simulink model "OMSv1_2x"  (Simulink 6.5)
settings: Solver=ode4  SolverMode=SingleTasking  StartTime=0.0  StopTime=5  FixedStep=0.001  MaxStep=0.001  RelTol=1e-3  AbsTol=1e-3
undefined symbols (not defined in the file): alexlaw, bs_onoff, bs_scale, bsfsacrit, bsfsvcrit, cnsgain, fs_onoff, fs_scale, fsdelaycalc, ltdrk, phasicgain, pmcgain, pmctau2, pmctau3, saccsw, spgain, tonicgain, tvrD, tvrN
libraries: simulink_extras x37
(part 3 of 5)

== system OMSv1_2x/OMS v1.2  07/21/05/IM CN-LMLN/Saccade Enable/prolong ==
  note: init Q = 0
  note: Stretch the duration of an input pulse, latching it at its value at pulse onset.
  note: The one integration step delay before the S&H block's S/H (bottom) input insures
      | that the input value to be latched is available to theS&H block's top input
      | before the S&H block tries to 'hold'.
  note: The start of the input pulse causes the value on input 1 to be held starting when the leading
      | edge occurs, and this value remains latched until 'delay' seconds after the pulse ends (trailing edge).
  note: 11/22/99
  note: init = 0
  note: init = 0
  value(in) : Inport
  " x/1000" : Constant  Orientation=up  Value=0.001
  Latch1 : simulink_extras/Flip Flops/S-R Flip-Flop  SystemSampleTime=-1  initial_condition=0
  Product : Product  SaturateOnIntegerOverflow=on  RndMeth=Zero  InputSameDT=on
  SampHold?2 : Subsystem
      mask Display: disp('S=L\nH=H')
  Terminator : Terminator
  Variable Transport Delay : VariableTransportDelay  MaximumDelay=10  MaximumPoints=prolong_buffersize
  leading edge detect : Subsystem
      mask Display: disp('Leading\nEdge Det')
  loop breaker2 : Memory
  stretch : Constant  Value=prolong
  trailing edge detect : Subsystem
      mask Display: disp('Trailing\nEdge Det')
  value(out) : Outport  InitialOutput=0
  wires:
  value(in)/1 -> leading edge detect/1(in_1), trailing edge detect/1(in_1), SampHold?2/1(Input)
  Variable Transport Delay/1 -> Latch1/2
  trailing edge detect/1(out_1) -> Variable Transport Delay/1
  leading edge detect/1(out_1) -> Latch1/1
  Latch1/1 -> loop breaker2/1
  SampHold?2/1(output) -> value(out)/1
  loop breaker2/1 -> SampHold?2/2(S/H?)
  stretch/1 -> Product/1
  Product/1 -> Variable Transport Delay/2
  " x/1000"/1 -> Product/2
  Latch1/2 -> Terminator/1

== system OMSv1_2x/OMS v1.2  07/21/05/IM CN-LMLN/Saccade Enable/trailing edge detect ==
  note: trailing edge detection
  note: It is also possible to remove the SIGNUM function
      | and the '==', and replace them with a simple
      | switch with a threshold of (say) 150 or so.
  PG : Inport
  Abs : Abs  SaturateOnIntegerOverflow=on
  Derivative : Derivative
  Relational Operator : RelationalOperator  Operator===  InputSameDT=on
  Sign : Signum
  Threshold 1 : Constant  Value=-1
  Latch R : Outport  InitialOutput=0
  wires:
  PG/1 -> Abs/1
  Relational Operator/1 -> Latch R/1
  Threshold 1/1 -> Relational Operator/2
  Sign/1 -> Relational Operator/1
  Derivative/1 -> Sign/1
  Abs/1 -> Derivative/1

== system OMSv1_2x/OMS v1.2  07/21/05/IM CN-LMLN/Saccade Motor Commmand/TCHNG Override ==
  note: (FF init state: Q=1)
  note: * Leading Edge of input ENABLEs output
  note: Operation:
  note: *FS Enabling is initially DISABLED
  note: * Output of TIMER circuit DISABLES output
  note: TCHNG Override
  "[tchng]" : Inport
  timer dur : Inport  Orientation=up  Port=2
  Latch1 : simulink_extras/Flip Flops/S-R Flip-Flop  SystemSampleTime=-1  initial_condition=1
  Terminator : Terminator
  event timer2 : Subsystem
      mask Display: disp('Event\nTimer2')
  leading edge detect : Subsystem
      mask Display: disp('Leading\nEdge Det')
  tchng sw : Outport  InitialOutput=0
  wires:
  "[tchng]"/1 -> leading edge detect/1(in_1), event timer2/1(_PG)
  timer dur/1 -> event timer2/2(_timer value (port))
  event timer2/1(out_1) -> Latch1/1
  leading edge detect/1(out_1) -> Latch1/2
  Latch1/1 -> tchng sw/1
  Latch1/2 -> Terminator/1

== system OMSv1_2x/OMS v1.2  07/21/05/IM CN-LMLN/Saccade Motor Commmand/Voluntary Saccade Switch ==
  note: Voluntary Saccade Switch
  note: move this outpt
      | to top switch
  note: last mod:
      | 02/26/01
  "[fphmag]" : Inport
  "[sacenab]" : Inport  Port=2
  "[fsorbs30]" : Inport  Port=3
  (0.5)1 : Switch  Threshold=.5  SaturateOnIntegerOverflow=on  InputSameDT=on
  (0.5)2 : Switch  Threshold=.5  SaturateOnIntegerOverflow=on  InputSameDT=on
  (0.5)3 : Switch  Threshold=.5  SaturateOnIntegerOverflow=on  InputSameDT=on
  Logical Operator4 : Logic  Operator=NOT  Inputs=1
  Logical Operator6 : Logic  Operator=OR
  oppose3 : Constant  Orientation=left  Value=0
  saccsw : Constant  Orientation=left  Value=saccsw
  "[vsmc]" : Outport  InitialOutput=0
  sacenab/0 : Outport  Port=2  InitialOutput=0
  wires:
  "[fphmag]"/1 -> (0.5)2/1
  "[fsorbs30]"/1 -> Logical Operator4/1
  Logical Operator4/1 -> Logical Operator6/2
  (0.5)2/1 -> (0.5)3/1
  Logical Operator6/1 -> sacenab/0/1
  saccsw/1 -> (0.5)2/3, (0.5)2/2, (0.5)1/2, (0.5)1/3
  "[sacenab]"/1 -> (0.5)1/1, (0.5)3/2
  (0.5)1/1 -> Logical Operator6/1
  oppose3/1 -> (0.5)3/3
  (0.5)3/1 -> "[vsmc]"/1

== system OMSv1_2x/OMS v1.2  07/21/05/IM CN-LMLN/Sampled Target Reconstruction/Boolify ==
  In1 : Inport
  Abs2 : Abs  SaturateOnIntegerOverflow=on
  direction1 : Signum
  Out1 : Outport  InitialOutput=0
  wires:
  direction1/1 -> Out1/1
  In1/1 -> Abs2/1
  Abs2/1 -> direction1/1

== system OMSv1_2x/OMS v1.2  07/21/05/IM CN-LMLN/Sampled Target Reconstruction/Boolify1 ==
  In1 : Inport
  Abs2 : Abs  SaturateOnIntegerOverflow=on
  direction1 : Signum
  Out1 : Outport  InitialOutput=0
  wires:
  Abs2/1 -> direction1/1
  In1/1 -> Abs2/1
  direction1/1 -> Out1/1

== system OMSv1_2x/OMS v1.2  07/21/05/IM CN-LMLN/Sampled Target Reconstruction/DZ 0.3 ==
  note: We just output zero when the dead zone is in effect, and leave the
      |  output alone the rest of the time.
  note: This block is a better implementation of a dead zone than  the
      | block supplied by SIMULINK, because here we don't _subtract_
      | the dead zone from the rest of output.
  in_1 : Inport
  Abs : Abs  Orientation=down  SaturateOnIntegerOverflow=on
  Relational Operator : RelationalOperator  InputSameDT=on
  Switch6 : Switch  Threshold=.5  SaturateOnIntegerOverflow=on  InputSameDT=on
  dead zone : Constant  Orientation=up  Value=.3
  pos (deg) criterion1 : Constant  Orientation=left  Value=0
  out_1 : Outport  InitialOutput=0
  wires:
  Relational Operator/1 -> Switch6/2
  dead zone/1 -> Relational Operator/2
  pos (deg) criterion1/1 -> Switch6/3
  Abs/1 -> Relational Operator/1
  in_1/1 -> Abs/1, Switch6/1
  Switch6/1 -> out_1/1

== system OMSv1_2x/OMS v1.2  07/21/05/IM CN-LMLN/Sampled Target Reconstruction/SampHold? ==
  note: When "S/H?" is HIGH, then "Input" is switched directly to the
      | output ("sample").  When "S/H?" is LOW, the current output is
      | maintained ("hold").
  Input : Inport
  S/H? : Inport  Port=2
  Memory : Memory  Orientation=left
  Sign : Signum
  Switch2 : Switch  Threshold=0.5  SaturateOnIntegerOverflow=on  InputSameDT=on
  output : Outport  InitialOutput=0
  wires:
  S/H?/1 -> Sign/1
  Sign/1 -> Switch2/2
  Input/1 -> Switch2/1
  Switch2/1 -> output/1, Memory/1
  Memory/1 -> Switch2/3

== system OMSv1_2x/OMS v1.2  07/21/05/IM CN-LMLN/Sampled Target Reconstruction/leading edge detect1 ==
  note: leading edge detection
  in_1 : Inport
  Abs : Abs  SaturateOnIntegerOverflow=on
  Derivative : Derivative
  Relational Operator : RelationalOperator  Operator===  InputSameDT=on
  Sign : Signum
  Threshold 1 : Constant
  out_1 : Outport  InitialOutput=0
  wires:
  Abs/1 -> Derivative/1
  Derivative/1 -> Sign/1
  Sign/1 -> Relational Operator/1
  Threshold 1/1 -> Relational Operator/2
  Relational Operator/1 -> out_1/1
  in_1/1 -> Abs/1

== system OMSv1_2x/OMS v1.2  07/21/05/IM CN-LMLN/Sampled Target Reconstruction/leading edge detect2 ==
  note: leading edge detection
  in_1 : Inport
  Abs : Abs  SaturateOnIntegerOverflow=on
  Derivative : Derivative
  Relational Operator : RelationalOperator  Operator===  InputSameDT=on
  Sign : Signum
  Threshold 1 : Constant
  out_1 : Outport  InitialOutput=0
  wires:
  in_1/1 -> Abs/1
  Relational Operator/1 -> out_1/1
  Threshold 1/1 -> Relational Operator/2
  Sign/1 -> Relational Operator/1
  Derivative/1 -> Sign/1
  Abs/1 -> Derivative/1

== system OMSv1_2x/OMS v1.2  07/21/05/IM CN-LMLN/Sampled Target Reconstruction/prolong ==
  note: init = 0
  note: init = 0
  note: 11/22/99
  note: The start of the input pulse causes the value on input 1 to be held starting when the leading
      | edge occurs, and this value remains latched until 'delay' seconds after the pulse ends (trailing edge).
  note: The one integration step delay before the S&H block's S/H (bottom) input insures
      | that the input value to be latched is available to theS&H block's top input
      | before the S&H block tries to 'hold'.
  note: Stretch the duration of an input pulse, latching it at its value at pulse onset.
  note: init Q = 0
  value(in) : Inport
  " x/1000" : Constant  Orientation=up  Value=0.001
  Latch1 : simulink_extras/Flip Flops/S-R Flip-Flop  SystemSampleTime=-1  initial_condition=0
  Product : Product  SaturateOnIntegerOverflow=on  RndMeth=Zero  InputSameDT=on
  SampHold?2 : Subsystem
      mask Display: disp('S=L\nH=H')
  Terminator : Terminator
  Variable Transport Delay : VariableTransportDelay  MaximumDelay=10  MaximumPoints=prolong_buffersize
  leading edge detect : Subsystem
      mask Display: disp('Leading\nEdge Det')
  loop breaker2 : Memory
  stretch : Constant  Value=prolong
  trailing edge detect : Subsystem
      mask Display: disp('Trailing\nEdge Det')
  value(out) : Outport  InitialOutput=0
  wires:
  " x/1000"/1 -> Product/2
  Product/1 -> Variable Transport Delay/2
  stretch/1 -> Product/1
  loop breaker2/1 -> SampHold?2/2(S/H?)
  SampHold?2/1(output) -> value(out)/1
  Latch1/1 -> loop breaker2/1
  leading edge detect/1(out_1) -> Latch1/1
  trailing edge detect/1(out_1) -> Variable Transport Delay/1
  Variable Transport Delay/1 -> Latch1/2
  value(in)/1 -> SampHold?2/1(Input), trailing edge detect/1(in_1), leading edge detect/1(in_1)
  Latch1/2 -> Terminator/1

== system OMSv1_2x/OMS v1.2  07/21/05/IM CN-LMLN/Sampled Target Reconstruction/prolong1 ==
  note: init Q = 0
  note: Stretch the duration of an input pulse, latching it at its value at pulse onset.
  note: The one integration step delay before the S&H block's S/H (bottom) input insures
      | that the input value to be latched is available to theS&H block's top input
      | before the S&H block tries to 'hold'.
  note: The start of the input pulse causes the value on input 1 to be held starting when the leading
      | edge occurs, and this value remains latched until 'delay' seconds after the pulse ends (trailing edge).
  note: 11/22/99
  note: init = 0
  note: init = 0
  value(in) : Inport
  " x/1000" : Constant  Orientation=up  Value=0.001
  Latch1 : simulink_extras/Flip Flops/S-R Flip-Flop  SystemSampleTime=-1  initial_condition=0
  Product : Product  SaturateOnIntegerOverflow=on  RndMeth=Zero  InputSameDT=on
  SampHold?2 : Subsystem
      mask Display: disp('S=L\nH=H')
  Terminator : Terminator
  Variable Transport Delay : VariableTransportDelay  MaximumDelay=10  MaximumPoints=prolong_buffersize
  leading edge detect : Subsystem
      mask Display: disp('Leading\nEdge Det')
  loop breaker2 : Memory
  stretch : Constant  Value=prolong
  trailing edge detect : Subsystem
      mask Display: disp('Trailing\nEdge Det')
  value(out) : Outport  InitialOutput=0
  wires:
  value(in)/1 -> leading edge detect/1(in_1), trailing edge detect/1(in_1), SampHold?2/1(Input)
  Variable Transport Delay/1 -> Latch1/2
  trailing edge detect/1(out_1) -> Variable Transport Delay/1
  leading edge detect/1(out_1) -> Latch1/1
  Latch1/1 -> loop breaker2/1
  SampHold?2/1(output) -> value(out)/1
  loop breaker2/1 -> SampHold?2/2(S/H?)
  stretch/1 -> Product/1
  Product/1 -> Variable Transport Delay/2
  " x/1000"/1 -> Product/2
  Latch1/2 -> Terminator/1

== system OMSv1_2x/OMS v1.2  07/21/05/IM CN-LMLN/Sampled Target Reconstruction/prolong2 ==
  note: init = 0
  note: init = 0
  note: 11/22/99
  note: The start of the input pulse causes the value on input 1 to be held starting when the leading
      | edge occurs, and this value remains latched until 'delay' seconds after the pulse ends (trailing edge).
  note: The one integration step delay before the S&H block's S/H (bottom) input insures
      | that the input value to be latched is available to theS&H block's top input
      | before the S&H block tries to 'hold'.
  note: Stretch the duration of an input pulse, latching it at its value at pulse onset.
  note: init Q = 0
  value(in) : Inport
  " x/1000" : Constant  Orientation=up  Value=0.001
  Latch1 : simulink_extras/Flip Flops/S-R Flip-Flop  SystemSampleTime=-1  initial_condition=0
  Product : Product  SaturateOnIntegerOverflow=on  RndMeth=Zero  InputSameDT=on
  SampHold?2 : Subsystem
      mask Display: disp('S=L\nH=H')
  Terminator : Terminator
  Variable Transport Delay : VariableTransportDelay  MaximumDelay=10  MaximumPoints=prolong_buffersize
  leading edge detect : Subsystem
      mask Display: disp('Leading\nEdge Det')
  loop breaker2 : Memory
  stretch : Constant  Value=prolong
  trailing edge detect : Subsystem
      mask Display: disp('Trailing\nEdge Det')
  value(out) : Outport  InitialOutput=0
  wires:
  " x/1000"/1 -> Product/2
  Product/1 -> Variable Transport Delay/2
  stretch/1 -> Product/1
  loop breaker2/1 -> SampHold?2/2(S/H?)
  SampHold?2/1(output) -> value(out)/1
  Latch1/1 -> loop breaker2/1
  leading edge detect/1(out_1) -> Latch1/1
  trailing edge detect/1(out_1) -> Variable Transport Delay/1
  Variable Transport Delay/1 -> Latch1/2
  value(in)/1 -> SampHold?2/1(Input), trailing edge detect/1(in_1), leading edge detect/1(in_1)
  Latch1/2 -> Terminator/1

== system OMSv1_2x/OMS v1.2  07/21/05/IM CN-LMLN/Slip Velocity Reconstruction/DZ 0.5 ==
  note: We just output zero when the dead zone is in effect, and leave the
      |  output alone the rest of the time.
  note: This block is a better implementation of a dead zone than  the
      | block supplied by SIMULINK, because here we don't _subtract_
      | the dead zone from the rest of output.
  in_1 : Inport
  in_2 : Inport  Port=2
  Abs : Abs  Orientation=down  SaturateOnIntegerOverflow=on
  Relational Operator : RelationalOperator  InputSameDT=on
  Switch6 : Switch  Threshold=.5  SaturateOnIntegerOverflow=on  InputSameDT=on
  pos (deg) criterion1 : Constant  Orientation=left  Value=0
  out_1 : Outport  InitialOutput=0
  wires:
  Relational Operator/1 -> Switch6/2
  pos (deg) criterion1/1 -> Switch6/3
  Switch6/1 -> out_1/1
  in_2/1 -> Relational Operator/2
  Abs/1 -> Relational Operator/1
  in_1/1 -> Abs/1, Switch6/1

== system OMSv1_2x/OMS v1.2  07/21/05/IM CN-LMLN/Slip Velocity Reconstruction/Lim 100 ==
  note: This block limits outputs to less than or equal to the "Limit" constant.
      | Inputs greater than "Limit" yield a zero output.
  in_1 : Inport
  Abs : Abs  SaturateOnIntegerOverflow=on
  Limit : Constant  Orientation=up  Value=100
  Product : Product  SaturateOnIntegerOverflow=on  RndMeth=Zero  InputSameDT=on
  Relational Operator : RelationalOperator  Operator=<=  InputSameDT=on
  out_1 : Outport  InitialOutput=0
  wires:
  in_1/1 -> Product/1, Abs/1
  Abs/1 -> Relational Operator/1
  Relational Operator/1 -> Product/2
  Limit/1 -> Relational Operator/2
  Product/1 -> out_1/1

== system OMSv1_2x/OMS v1.2  07/21/05/IM CN-LMLN/Slip Velocity Reconstruction/SampHold?4 ==
  note: When "S/H?" is HIGH, then "Input" is switched directly to the
      | output ("sample").  When "S/H?" is LOW, the current output is
      | maintained ("hold").
  Input : Inport
  S/H? : Inport  Port=2
  Memory : Memory  Orientation=left
  Sign : Signum
  Switch2 : Switch  Threshold=0.5  SaturateOnIntegerOverflow=on  InputSameDT=on
  output : Outport  InitialOutput=0
  wires:
  S/H?/1 -> Sign/1
  Sign/1 -> Switch2/2
  Switch2/1 -> output/1, Memory/1
  Input/1 -> Switch2/1
  Memory/1 -> Switch2/3

== system OMSv1_2x/OMS v1.2  07/21/05/PG w rNI1/PW funct/Good Reset Integrator1 ==
  note: This Resettable integrator won't (incorrectly) integrate the input even
      | when the reset signal is held, unlike the SIMULINK RI, which
      | gives a one time-step error.
  note: reset on either rising
      | edge or level signal
  note: changed 7/22
  note: Using 'state' port, rather than 'output'
      | port to avoid algebraic loop*
  note: *see: www.mathworks.com/access/helpdesk/toolbox/simulink/slref/integrator.html
  input : Inport
  reset? : Inport  Port=2
  initial condition : Inport  Port=3
  Integrator : Integrator  ExternalReset=either  InitialConditionSource=external  ShowStatePort=on
  Logical Operator2 : Logic  Orientation=up  Operator=NOT  Inputs=1
  Product : Product  SaturateOnIntegerOverflow=on  RndMeth=Zero  InputSameDT=on
  Terminator : Terminator
  out_1 : Outport  InitialOutput=0
  wires:
  initial condition/1 -> Integrator/3
  Logical Operator2/1 -> Product/2
  input/1 -> Product/1
  Product/1 -> Integrator/1
  reset?/1 -> Integrator/2, Logical Operator2/1
  Integrator/State -> out_1/1
  Integrator/1 -> Terminator/1

== system OMSv1_2x/OMS v1.2  07/21/05/PG w rNI1/PW funct/Input Switch ==
  mcspl : Inport
  pgw : Inport  Port=2
  Switch2 : Switch  Threshold=0.5  SaturateOnIntegerOverflow=on  InputSameDT=on
  lead/trail edge det : Subsystem
      mask Display: disp('Lead/Trail\nEdge Det')
  mcsw : Outport  InitialOutput=0
  wires:
  mcspl/1 -> Switch2/1, lead/trail edge det/1(in_1)
  pgw/1 -> Switch2/2
  lead/trail edge det/1(out_1) -> Switch2/3
  Switch2/1 -> mcsw/1

== system OMSv1_2x/OMS v1.2  07/21/05/PG w rNI1/RefLatch (Default = 50ms)/trailing edge ==
  note: (FF init state: Q=1)
  note: (Init input: 0)
  note: When the latency period is over, the block is again ENABLED.  ONLY once the latency period is
      | over does the block accept any new input.  (i.e. any input that occurs during the disabled
      |  latency period is ignored)
  note: When input occurs, the block then becomes DISABLED, and remains so for the
      | duration of the latency period (set either via the mask, or by setting "delay" from the command line)
  note: Block operation: it is initially ENABLED, allowing input.
  note: latency period starts with the END of the pulse, rather than the beginning.
  note: (Init input: 1)
  note: (Must see a trailing edge from the
      | signal AS WELL)
  note: This upper branch prevents response
      | to transients caused by the switch
      | toggling states
  in_1 : Inport
  Logical Operator : Logic
  S-R Flip-Flop : simulink_extras/Flip Flops/S-R Flip-Flop  SystemSampleTime=-1  initial_condition=1
  Switch1 : Switch  Threshold=.5  SaturateOnIntegerOverflow=on  InputSameDT=on
  Terminator : Terminator
  Threshold 3 : Constant  Orientation=left  Value=0
  loop breaker : Memory  Orientation=left  X0=1
  refractory period : TransportDelay  DelayTime=(delay)/1000
  trailing edge det : Subsystem
      mask Display: disp('Trailing\nEdge Det')
  trailing edge det1 : Subsystem
      mask Display: disp('Trailing\nEdge Det')
  out_1 : Outport  InitialOutput=0
  wires:
  S-R Flip-Flop/1 -> out_1/1, loop breaker/1
  Logical Operator/1 -> S-R Flip-Flop/2, refractory period/1
  trailing edge det/1(out_1) -> Logical Operator/1
  trailing edge det1/1(out_1) -> Logical Operator/2
  in_1/1 -> Switch1/1, trailing edge det/1(in_1)
  refractory period/1 -> S-R Flip-Flop/1
  loop breaker/1 -> Switch1/2
  Threshold 3/1 -> Switch1/3
  Switch1/1 -> trailing edge det1/1(in_1)
  S-R Flip-Flop/2 -> Terminator/1

== system OMSv1_2x/OMS v1.2  07/21/05/IM CN-LMLN/BS/FS Logic/BS Enable1/BS Timing ==
  note: (FF init state: Q=0)
  note: * Leading Edge of input ENABLEs output
  note: Operation:
  note: *BS Enabling is initially DISABLED
  note: * Output of TIMER circuit DISABLES output
  note: BS Timing
  From  <= [cmpr] : Inport
  timer dur : Inport  Orientation=up  Port=2
  Latch1 : simulink_extras/Flip Flops/S-R Flip-Flop  SystemSampleTime=-1  initial_condition=0
  Terminator : Terminator
  event timer2 : Subsystem
      mask Display: disp('Event\nTimer2')
  leading edge detect : Subsystem
      mask Display: disp('Leading\nEdge Det')
  "[bsenab]" : Outport  InitialOutput=0
  wires:
  From  <= [cmpr]/1 -> leading edge detect/1(in_1), event timer2/1(_PG)
  leading edge detect/1(out_1) -> Latch1/1
  event timer2/1(out_1) -> Latch1/2
  Latch1/1 -> "[bsenab]"/1
  timer dur/1 -> event timer2/2(_timer value (port))
  Latch1/2 -> Terminator/1

== system OMSv1_2x/OMS v1.2  07/21/05/IM CN-LMLN/BS/FS Logic/FS Enable/FS Timing ==
  note: FS Timing
  note: * Output of TIMER circuit DISABLES output
  note: *FS Enabling is initially DISABLED
  note: Operation:
  note: * Leading Edge of input ENABLEs output
  note: (FF init state: Q=0)
  From  <= [cmpr] : Inport
  timer dur : Inport  Orientation=up  Port=2
  Latch1 : simulink_extras/Flip Flops/S-R Flip-Flop  SystemSampleTime=-1  initial_condition=0
  Terminator : Terminator
  event timer2 : Subsystem
      mask Display: disp('Event\nTimer2')
  leading edge detect : Subsystem
      mask Display: disp('Leading\nEdge Det')
  "[fsenab]" : Outport  InitialOutput=0
  wires:
  timer dur/1 -> event timer2/2(_timer value (port))
  Latch1/1 -> "[fsenab]"/1
  event timer2/1(out_1) -> Latch1/2
  leading edge detect/1(out_1) -> Latch1/1
  From  <= [cmpr]/1 -> event timer2/1(_PG), leading edge detect/1(in_1)
  Latch1/2 -> Terminator/1

== system OMSv1_2x/OMS v1.2  07/21/05/IM CN-LMLN/BS/FS Logic/FS Enable/SampHold?1 ==
  note: When "S/H?" is LOW, then "Input" is switched directly to the
      | output ("sample").  When "S/H?" is HIGH, the current output is
      | maintained ("hold").
  Input : Inport
  S/H? : Inport  Port=2
  Memory : Memory  Orientation=left
  Sign : Signum
  Switch2 : Switch  Threshold=0.5  SaturateOnIntegerOverflow=on  InputSameDT=on
  output : Outport  InitialOutput=0
  wires:
  Input/1 -> Switch2/3
  Memory/1 -> Switch2/1
  S/H?/1 -> Sign/1
  Sign/1 -> Switch2/2
  Switch2/1 -> output/1, Memory/1

== system OMSv1_2x/OMS v1.2  07/21/05/IM CN-LMLN/BS/FS Logic/FS or BS?/Boolify ==
  In1 : Inport
  Abs2 : Abs  SaturateOnIntegerOverflow=on
  direction1 : Signum
  Out1 : Outport  InitialOutput=0
  wires:
  Abs2/1 -> direction1/1
  In1/1 -> Abs2/1
  direction1/1 -> Out1/1

== system OMSv1_2x/OMS v1.2  07/21/05/IM CN-LMLN/BS/FS Logic/FS or BS?/SampHold?1 ==
  note: When "S/H?" is LOW, then "Input" is switched directly to the
      | output ("sample").  When "S/H?" is HIGH, the current output is
      | maintained ("hold").
  Input : Inport
  S/H? : Inport  Port=2
  Memory : Memory  Orientation=left
  Sign : Signum
  Switch2 : Switch  Threshold=0.5  SaturateOnIntegerOverflow=on  InputSameDT=on
  output : Outport  InitialOutput=0
  wires:
  Input/1 -> Switch2/3
  Memory/1 -> Switch2/1
  S/H?/1 -> Sign/1
  Sign/1 -> Switch2/2
  Switch2/1 -> output/1, Memory/1

== system OMSv1_2x/OMS v1.2  07/21/05/IM CN-LMLN/BS/FS Logic/TCHNG Override/event timer2 ==
  note: In 2) Subsequent events DO NOT reset the counter; it only resets when it
      | reaches zero
  note: 2) A new event (leading or trailing edge) is detected. -- Only case 1)
  note: 1) The count reaches its limit (set in "timer value") -- Both case 1) and 2)
  note: In 1), Any event (leading or trailing edge) will reset the counter so that it
      | counts down from the end trailing edge) of that event.
  note: It has TWO modes: 1) Event resettable and 2) Event Non-resettable
  note: The real trick here is understanding how to reload the countdown.
      | It resets if either of two conditions is met:
  note: The "OR" gate allows either of these conditions to reset the circuit.  The delay before the
      | "S" input of the flip-flop prevents both "S" and "R" from being set simultaneously, because
      | this would put the flip-flop in an undefined state.
  note: Therefore, an event first RESETS and then SETS the flip-flop.
  note: (Init input: 0)
  note: (FF init state: Q=0)
  note: (Init input: 0)
  note: This block is an RESETTABLE EVENT TIMER.  It outputs a spike of unit height xx milliseconds
      | (set by "timer value") after it detects an event ( i.e a TRAILING edge which represents the end of a
      |  saccadic pulse)
  note: Resettable
      | Event Timer
  _PG : Inport
  _timer value (port) : Inport  Port=2
  1 msec : TransportDelay  DelayTime=.001
  Clock : Clock
      settings: Decimation=10
  Latch1 : simulink_extras/Flip Flops/S-R Flip-Flop  SystemSampleTime=-1  initial_condition=0
  Logical Operator : Logic  Operator=OR  Inputs=3
  Logical Operator1 : Logic
  Logical Operator2 : Logic
  Relational Operator : RelationalOperator  InputSameDT=on
  SampHold?1 : Subsystem
      mask Display: disp('S&H\n(S=L)\n(H=H)')
  Sum : Sum  Inputs=+-  SaturateOnIntegerOverflow=on  InputSameDT=on
  Terminator : Terminator
  event resettable? : Constant  Orientation=up  Value=0
  leading edge detect : Subsystem
      mask Display: disp('Leading\nEdge Det')
  loop breaker : Memory  Orientation=left
  trailing edge detect : Subsystem
      mask Display: disp('Trailing\nEdge Det')
  out_1 : Outport  InitialOutput=0
  wires:
  event resettable?/1 -> Logical Operator2/2, Logical Operator1/2
  leading edge detect/1(out_1) -> Logical Operator2/1
  Logical Operator2/1 -> Logical Operator/2
  trailing edge detect/1(out_1) -> Logical Operator1/1, 1 msec/1
  Logical Operator1/1 -> Logical Operator/1
  loop breaker/1 -> Logical Operator/3
  _PG/1 -> leading edge detect/1(in_1), trailing edge detect/1(in_1)
  Latch1/1 -> SampHold?1/2(S/H?)
  Relational Operator/1 -> out_1/1, loop breaker/1
  Sum/1 -> Relational Operator/1
  Clock/1 -> Sum/1, SampHold?1/1(Input)
  SampHold?1/1(output) -> Sum/2
  Logical Operator/1 -> Latch1/2
  1 msec/1 -> Latch1/1
  _timer value (port)/1 -> Relational Operator/2
  Latch1/2 -> Terminator/1

== system OMSv1_2x/OMS v1.2  07/21/05/IM CN-LMLN/BS/FS Logic/TCHNG Override/leading edge detect ==
  note: leading edge detection
  in_1 : Inport
  Abs : Abs  SaturateOnIntegerOverflow=on
  Derivative : Derivative
  Relational Operator : RelationalOperator  Operator===  InputSameDT=on
  Sign : Signum
  Threshold 1 : Constant
  out_1 : Outport  InitialOutput=0
  wires:
  in_1/1 -> Abs/1
  Relational Operator/1 -> out_1/1
  Threshold 1/1 -> Relational Operator/2
  Sign/1 -> Relational Operator/1
  Derivative/1 -> Sign/1
  Abs/1 -> Derivative/1

== system OMSv1_2x/OMS v1.2  07/21/05/IM CN-LMLN/BS/FS Logic/prolong/SampHold?2 ==
  note: When "S/H?" is LOW, then "Input" is switched directly to the
      | output ("sample").  When "S/H?" is HIGH, the current output is
      | maintained ("hold").
  Input : Inport
  S/H? : Inport  Port=2
  Memory : Memory  Orientation=left
  Sign : Signum
  Switch2 : Switch  Threshold=0.5  SaturateOnIntegerOverflow=on  InputSameDT=on
  output : Outport  InitialOutput=0
  wires:
  S/H?/1 -> Sign/1
  Sign/1 -> Switch2/2
  Input/1 -> Switch2/3
  Switch2/1 -> Memory/1, output/1
  Memory/1 -> Switch2/1

== system OMSv1_2x/OMS v1.2  07/21/05/IM CN-LMLN/BS/FS Logic/prolong/leading edge detect ==
  note: leading edge detection
  in_1 : Inport
  Abs : Abs  SaturateOnIntegerOverflow=on
  Derivative : Derivative
  Relational Operator : RelationalOperator  Operator===  InputSameDT=on
  Sign : Signum
  Threshold 1 : Constant
  out_1 : Outport  InitialOutput=0
  wires:
  in_1/1 -> Abs/1
  Relational Operator/1 -> out_1/1
  Threshold 1/1 -> Relational Operator/2
  Sign/1 -> Relational Operator/1
  Derivative/1 -> Sign/1
  Abs/1 -> Derivative/1

== system OMSv1_2x/OMS v1.2  07/21/05/IM CN-LMLN/BS/FS Logic/prolong/trailing edge detect ==
  note: It is also possible to remove the SIGNUM function
      | and the '==', and replace them with a simple
      | switch with a threshold of (say) 150 or so.
  note: trailing edge detection
  in_1 : Inport
  Abs : Abs  SaturateOnIntegerOverflow=on
  Derivative : Derivative
  Relational Operator : RelationalOperator  Operator===  InputSameDT=on
  Sign : Signum
  Threshold 1 : Constant  Value=-1
  out_1 : Outport  InitialOutput=0
  wires:
  Abs/1 -> Derivative/1
  Derivative/1 -> Sign/1
  Sign/1 -> Relational Operator/1
  Threshold 1/1 -> Relational Operator/2
  Relational Operator/1 -> out_1/1
  in_1/1 -> Abs/1

== system OMSv1_2x/OMS v1.2  07/21/05/IM CN-LMLN/MdlPlnt+/OMN2/SampHold? ==
  note: When "S/H?" is LOW, then "Input" is switched directly to the
      | output ("sample").  When "S/H?" is HIGH, the current output is
      | maintained ("hold").
  Input : Inport
  S/H? : Inport  Port=2
  Memory : Memory  Orientation=left
  Sign : Signum
  Switch2 : Switch  Threshold=0.5  SaturateOnIntegerOverflow=on  InputSameDT=on
  output : Outport  InitialOutput=0
  wires:
  Switch2/1 -> Memory/1, output/1
  Sign/1 -> Switch2/2
  Input/1 -> Switch2/3
  S/H?/1 -> Sign/1
  Memory/1 -> Switch2/1

== system OMSv1_2x/OMS v1.2  07/21/05/IM CN-LMLN/Sacc Blank/event timer1/SampHold?1 ==
  note: When "S/H?" is LOW, then "Input" is switched directly to the
      | output ("sample").  When "S/H?" is HIGH, the current output is
      | maintained ("hold").
  Input : Inport
  S/H? : Inport  Port=2
  Memory : Memory  Orientation=left
  Sign : Signum
  Switch2 : Switch  Threshold=0.5  SaturateOnIntegerOverflow=on  InputSameDT=on
  output : Outport  InitialOutput=0
  wires:
  Switch2/1 -> Memory/1, output/1
  Sign/1 -> Switch2/2
  S/H?/1 -> Sign/1
  Memory/1 -> Switch2/1
  Input/1 -> Switch2/3

== system OMSv1_2x/OMS v1.2  07/21/05/IM CN-LMLN/Sacc Blank/event timer1/leading edge detect ==
  note: It is also possible to remove the SIGNUM function
      | and the '==', and replace them with a simple
      | switch with a threshold of (say) 150 or so.
  note: leading edge detection
  in_1 : Inport
  Abs : Abs  SaturateOnIntegerOverflow=on
  Derivative : Derivative
  Relational Operator : RelationalOperator  Operator===  InputSameDT=on
  Sign : Signum
  Threshold 1 : Constant
  out_1 : Outport  InitialOutput=0
  wires:
  Abs/1 -> Derivative/1
  Derivative/1 -> Sign/1
  Sign/1 -> Relational Operator/1
  Threshold 1/1 -> Relational Operator/2
  Relational Operator/1 -> out_1/1
  in_1/1 -> Abs/1

== system OMSv1_2x/OMS v1.2  07/21/05/IM CN-LMLN/Sacc Blank/event timer1/trailing edge detect ==
  note: trailing edge detection
  note: It is also possible to remove the SIGNUM function
      | and the '==', and replace them with a simple
      | switch with a threshold of (say) 150 or so.
  in_1 : Inport
  Abs : Abs  SaturateOnIntegerOverflow=on
  Derivative : Derivative
  Relational Operator : RelationalOperator  Operator===  InputSameDT=on
  Sign : Signum
  Threshold 1 : Constant  Value=-1
  out_1 : Outport  InitialOutput=0
  wires:
  in_1/1 -> Abs/1
  Relational Operator/1 -> out_1/1
  Threshold 1/1 -> Relational Operator/2
  Sign/1 -> Relational Operator/1
  Derivative/1 -> Sign/1
  Abs/1 -> Derivative/1

== system OMSv1_2x/OMS v1.2  07/21/05/IM CN-LMLN/Saccade Enable/Enable Control/2 ms ==
  note: init Q = 0
  note: Stretch the duration of an input pulse, latching it at its value at pulse onset.
  note: The one integration step delay before the S&H block's S/H (bottom) input insures
      | that the input value to be latched is available to theS&H block's top input
      | before the S&H block tries to 'hold'.
  note: The start of the input pulse causes the value on input 1 to be held starting when the leading
      | edge occurs, and this value remains latched until 'delay' seconds after the pulse ends (trailing edge).
  note: 11/22/99
  note: init = 0
  note: init = 0
  value(in) : Inport
  " x/1000" : Constant  Orientation=up  Value=0.001
  Latch1 : simulink_extras/Flip Flops/S-R Flip-Flop  SystemSampleTime=-1  initial_condition=0
  Product : Product  SaturateOnIntegerOverflow=on  RndMeth=Zero  InputSameDT=on
  SampHold?2 : Subsystem
      mask Display: disp('S=L\nH=H')
  Terminator : Terminator
  Variable Transport Delay : VariableTransportDelay  MaximumDelay=10  MaximumPoints=prolong_buffersize
  leading edge detect : Subsystem
      mask Display: disp('Leading\nEdge Det')
  loop breaker2 : Memory
  stretch : Constant  Value=prolong
  trailing edge detect : Subsystem
      mask Display: disp('Trailing\nEdge Det')
  value(out) : Outport  InitialOutput=0
  wires:
  value(in)/1 -> leading edge detect/1(in_1), trailing edge detect/1(in_1), SampHold?2/1(Input)
  Variable Transport Delay/1 -> Latch1/2
  trailing edge detect/1(out_1) -> Variable Transport Delay/1
  leading edge detect/1(out_1) -> Latch1/1
  Latch1/1 -> loop breaker2/1
  SampHold?2/1(output) -> value(out)/1
  loop breaker2/1 -> SampHold?2/2(S/H?)
  stretch/1 -> Product/1
  Product/1 -> Variable Transport Delay/2
  " x/1000"/1 -> Product/2
  Latch1/2 -> Terminator/1

== system OMSv1_2x/OMS v1.2  07/21/05/IM CN-LMLN/Saccade Enable/Enable Control/50 ms ==
  note: init = 0
  note: init = 0
  note: 11/22/99
  note: The start of the input pulse causes the value on input 1 to be held starting when the leading
      | edge occurs, and this value remains latched until 'delay' seconds after the pulse ends (trailing edge).
  note: The one integration step delay before the S&H block's S/H (bottom) input insures
      | that the input value to be latched is available to theS&H block's top input
      | before the S&H block tries to 'hold'.
  note: Stretch the duration of an input pulse, latching it at its value at pulse onset.
  note: init Q = 0
  value(in) : Inport
  " x/1000" : Constant  Orientation=up  Value=0.001
  Latch1 : simulink_extras/Flip Flops/S-R Flip-Flop  SystemSampleTime=-1  initial_condition=0
  Product : Product  SaturateOnIntegerOverflow=on  RndMeth=Zero  InputSameDT=on
  SampHold?2 : Subsystem
      mask Display: disp('S=L\nH=H')
  Terminator : Terminator
  Variable Transport Delay : VariableTransportDelay  MaximumDelay=10  MaximumPoints=prolong_buffersize
  leading edge detect : Subsystem
      mask Display: disp('Leading\nEdge Det')
  loop breaker2 : Memory
  stretch : Constant  Value=prolong
  trailing edge detect : Subsystem
      mask Display: disp('Trailing\nEdge Det')
  value(out) : Outport  InitialOutput=0
  wires:
  " x/1000"/1 -> Product/2
  Product/1 -> Variable Transport Delay/2
  stretch/1 -> Product/1
  loop breaker2/1 -> SampHold?2/2(S/H?)
  SampHold?2/1(output) -> value(out)/1
  Latch1/1 -> loop breaker2/1
  leading edge detect/1(out_1) -> Latch1/1
  trailing edge detect/1(out_1) -> Variable Transport Delay/1
  Variable Transport Delay/1 -> Latch1/2
  value(in)/1 -> SampHold?2/1(Input), trailing edge detect/1(in_1), leading edge detect/1(in_1)
  Latch1/2 -> Terminator/1

== system OMSv1_2x/OMS v1.2  07/21/05/IM CN-LMLN/Saccade Enable/Enable Control/Boolify ==
  In1 : Inport
  Abs2 : Abs  SaturateOnIntegerOverflow=on
  direction1 : Signum
  Out1 : Outport  InitialOutput=0
  wires:
  Abs2/1 -> direction1/1
  In1/1 -> Abs2/1
  direction1/1 -> Out1/1

== system OMSv1_2x/OMS v1.2  07/21/05/IM CN-LMLN/Saccade Enable/Enable Control/Boolify1 ==
  In1 : Inport
  Abs2 : Abs  SaturateOnIntegerOverflow=on
  direction1 : Signum
  Out1 : Outport  InitialOutput=0
  wires:
  Abs2/1 -> direction1/1
  In1/1 -> Abs2/1
  direction1/1 -> Out1/1

== system OMSv1_2x/OMS v1.2  07/21/05/IM CN-LMLN/Saccade Enable/Enable Control/Boolify2 ==
  In1 : Inport
  Abs2 : Abs  SaturateOnIntegerOverflow=on
  direction1 : Signum
  Out1 : Outport  InitialOutput=0
  wires:
  Abs2/1 -> direction1/1
  In1/1 -> Abs2/1
  direction1/1 -> Out1/1

== system OMSv1_2x/OMS v1.2  07/21/05/IM CN-LMLN/Saccade Enable/Enable Control/ECPY Timing ==
  note: ECPY Timing
  note: (Init input:0)
  note: (Init input: 1)
  note: (FF init state: Q=0)
  note: (Init input: 0)
  note: (FF init state: Q=0)
  note: (((see original refract latch block for full description of operation.)))
  note: This signal is used by the Internal Monitor to decide when to compare EFERENCE COPY eye position with old eye position to decide if an appropriate saccade was made.
  note: This block outputs an ENABLE signal xx milliseconds long (set in "enable duration"), starting xx milliseconds (set in "post-pulse delay time") AFTER the input pulse concludes.
  note: If the FF init state is 0, then the block's initial output will be zero. If the FF init state is 1, then the block's initial output will be one.
  note: Corrective Saccades
  ECPY EnCntr [ecenctrl] : Inport
  Latch2 : simulink_extras/Flip Flops/S-R Flip-Flop  SystemSampleTime=-1  initial_condition=0
  Latch4 : simulink_extras/Flip Flops/S-R Flip-Flop  SystemSampleTime=-1  initial_condition=0
  Switch1 : Switch  Threshold=.5  SaturateOnIntegerOverflow=on  InputSameDT=on
  Terminator : Terminator
  Threshold 3 : Constant  Orientation=left  Value=0
  enab dur 10ms : TransportDelay  DelayTime=.01  InitialOutput=1
  leading edge detect : Subsystem
      mask Display: disp('Leading\nEdge Det')
  leading edge detect1 : Subsystem
      mask Display: disp('Leading\nEdge Det')
  loop breaker : Memory  Orientation=left
  or : Logic  Operator=OR
  post-pulse delay 130ms : TransportDelay  DelayTime=.13
  trailing edge detect : Subsystem
      mask Display: disp('Trailing\nEdge Det')
  ECPY Enable [ecpyenab] : Outport  InitialOutput=0
  wires:
  or/1 -> Latch4/2
  trailing edge detect/1(out_1) -> or/1, post-pulse delay 130ms/1
  Switch1/1 -> leading edge detect1/1(in_1), trailing edge detect/1(in_1)
  leading edge detect1/1(out_1) -> or/2
  ECPY EnCntr [ecenctrl]/1 -> Switch1/1
  Threshold 3/1 -> Switch1/3
  loop breaker/1 -> Switch1/2
  Latch2/1 -> ECPY Enable [ecpyenab]/1
  leading edge detect/1(out_1) -> enab dur 10ms/1, Latch2/1
  enab dur 10ms/1 -> Latch2/2
  Latch2/2 -> loop breaker/1
  post-pulse delay 130ms/1 -> Latch4/1
  Latch4/1 -> leading edge detect/1(in_1)
  Latch4/2 -> Terminator/1

== system OMSv1_2x/OMS v1.2  07/21/05/IM CN-LMLN/Saccade Enable/Enable Control/event timer1 ==
  note: Resettable
      | Event Timer
  note: This block is an RESETTABLE EVENT TIMER.  It outputs a spike of unit height xx milliseconds
      | (set by "timer value") after it detects an event ( i.e a TRAILING edge which represents the end of a
      |  saccadic pulse)
  note: (Init input: 0)
  note: (FF init state: Q=0)
  note: (Init input: 0)
  note: Therefore, an event first RESETS and then SETS the flip-flop.
  note: The "OR" gate allows either of these conditions to reset the circuit.  The delay before the
      | "S" input of the flip-flop prevents both "S" and "R" from being set simultaneously, because
      | this would put the flip-flop in an undefined state.
  note: The real trick here is understanding how to reload the countdown.
      | It resets if either of two conditions is met:
  note: It has TWO modes: 1) Event resettable and 2) Event Non-resettable
  note: In 1), Any event (leading or trailing edge) will reset the counter so that it
      | counts down from the end trailing edge) of that event.
  note: 1) The count reaches its limit (set in "timer value") -- Both case 1) and 2)
  note: 2) A new event (leading or trailing edge) is detected. -- Only case 1)
  note: In 2) Subsequent events DO NOT reset the counter; it only resets when it
      | reaches zero
  SW out : Inport
  _timer value (port) : Inport  Port=2
  1 msec : TransportDelay  DelayTime=.001
  Clock : Clock
      settings: Decimation=10
  Latch1 : simulink_extras/Flip Flops/S-R Flip-Flop  SystemSampleTime=-1  initial_condition=0
  Logical Operator : Logic  Operator=OR  Inputs=3
  Logical Operator1 : Logic
  Logical Operator2 : Logic
  Relational Operator : RelationalOperator  InputSameDT=on
  SampHold?1 : Subsystem
      mask Display: disp('S&H\n(S=L)\n(H=H)')
  Sum : Sum  Inputs=+-  SaturateOnIntegerOverflow=on  InputSameDT=on
  Terminator : Terminator
  event resettable? : Constant  Orientation=up
  leading edge detect : Subsystem
      mask Display: disp('Leading\nEdge Det')
  loop breaker : Memory  Orientation=left
  trailing edge detect : Subsystem
      mask Display: disp('Trailing\nEdge Det')
  FF Reset : Outport  InitialOutput=0
  wires:
  _timer value (port)/1 -> Relational Operator/2
  1 msec/1 -> Latch1/1
  Logical Operator/1 -> Latch1/2
  SampHold?1/1(output) -> Sum/2
  Relational Operator/1 -> loop breaker/1, FF Reset/1
  SW out/1 -> trailing edge detect/1(in_1), leading edge detect/1(in_1)
  Clock/1 -> Sum/1, SampHold?1/1(Input)
  Sum/1 -> Relational Operator/1
  Latch1/1 -> SampHold?1/2(S/H?)
  loop breaker/1 -> Logical Operator/3
  Logical Operator1/1 -> Logical Operator/1
  trailing edge detect/1(out_1) -> Logical Operator1/1, 1 msec/1
  Logical Operator2/1 -> Logical Operator/2
  leading edge detect/1(out_1) -> Logical Operator2/1
  event resettable?/1 -> Logical Operator2/2, Logical Operator1/2
  Latch1/2 -> Terminator/1

== system OMSv1_2x/OMS v1.2  07/21/05/IM CN-LMLN/Saccade Enable/Enable Control/leading edge detect ==
  note: It is also possible to remove the SIGNUM function
      | and the '==', and replace them with a simple
      | switch with a threshold of (say) 150 or so.
  note: leading edge detection
  in_1 : Inport
  Abs : Abs  SaturateOnIntegerOverflow=on
  Derivative : Derivative
  Relational Operator : RelationalOperator  Operator===  InputSameDT=on
  Sign : Signum
  Threshold 1 : Constant
  out_1 : Outport  InitialOutput=0
  wires:
  Abs/1 -> Derivative/1
  Derivative/1 -> Sign/1
  Sign/1 -> Relational Operator/1
  Threshold 1/1 -> Relational Operator/2
  Relational Operator/1 -> out_1/1
  in_1/1 -> Abs/1

== system OMSv1_2x/OMS v1.2  07/21/05/IM CN-LMLN/Saccade Enable/Enable Control/leading edge detect2 ==
  note: leading edge detection
  note: It is also possible to remove the SIGNUM function
      | and the '==', and replace them with a simple
      | switch with a threshold of (say) 150 or so.
  in_1 : Inport
  Abs : Abs  SaturateOnIntegerOverflow=on
  Derivative : Derivative
  Relational Operator : RelationalOperator  Operator===  InputSameDT=on
  Sign : Signum
  Threshold 1 : Constant
  out_1 : Outport  InitialOutput=0
  wires:
  in_1/1 -> Abs/1
  Relational Operator/1 -> out_1/1
  Threshold 1/1 -> Relational Operator/2
  Sign/1 -> Relational Operator/1
  Derivative/1 -> Sign/1
  Abs/1 -> Derivative/1

== system OMSv1_2x/OMS v1.2  07/21/05/IM CN-LMLN/Saccade Enable/Enable Control/trailing edge detect ==
  note: It is also possible to remove the SIGNUM function
      | and the '==', and replace them with a simple
      | switch with a threshold of (say) 150 or so.
  note: trailing edge detection
  PG : Inport
  Abs : Abs  SaturateOnIntegerOverflow=on
  Derivative : Derivative
  Relational Operator : RelationalOperator  Operator===  InputSameDT=on
  Sign : Signum
  Threshold 1 : Constant  Value=-1
  Latch R : Outport  InitialOutput=0
  wires:
  Abs/1 -> Derivative/1
  Derivative/1 -> Sign/1
  Sign/1 -> Relational Operator/1
  Threshold 1/1 -> Relational Operator/2
  Relational Operator/1 -> Latch R/1
  PG/1 -> Abs/1

== system OMSv1_2x/OMS v1.2  07/21/05/IM CN-LMLN/Saccade Enable/LN FPh Gen/DZ 4 ==
  note: This block is a better implementation of a dead zone than  the
      | block supplied by SIMULINK, because here we don't _subtract_
      | the dead zone from the rest of output.
  note: We just output zero when the dead zone is in effect, and leave the
      |  output alone the rest of the time.
  in_1 : Inport
  Abs : Abs  Orientation=down  SaturateOnIntegerOverflow=on
  Relational Operator : RelationalOperator  InputSameDT=on
  Switch6 : Switch  Threshold=.5  SaturateOnIntegerOverflow=on  InputSameDT=on
  dead zone : Constant  Orientation=up  Value=4
  pos (deg) criterion1 : Constant  Orientation=left  Value=0
  out_1 : Outport  InitialOutput=0
  wires:
  Switch6/1 -> out_1/1
  in_1/1 -> Switch6/1, Abs/1
  Abs/1 -> Relational Operator/1
  pos (deg) criterion1/1 -> Switch6/3
  dead zone/1 -> Relational Operator/2
  Relational Operator/1 -> Switch6/2

== system OMSv1_2x/OMS v1.2  07/21/05/IM CN-LMLN/Saccade Enable/LN FPh Gen/SampHold?1 ==
  note: When "S/H?" is HIGH, then "Input" is switched directly to the
      | output ("sample").  When "S/H?" is LOW, the current output is
      | maintained ("hold").
  Input : Inport
  S/H? : Inport  Port=2
  Memory : Memory  Orientation=left
  Sign : Signum
  Switch2 : Switch  Threshold=0.5  SaturateOnIntegerOverflow=on  InputSameDT=on
  output : Outport  InitialOutput=0
  wires:
  Memory/1 -> Switch2/3
  Input/1 -> Switch2/1
  Switch2/1 -> Memory/1, output/1
  Sign/1 -> Switch2/2
  S/H?/1 -> Sign/1

== system OMSv1_2x/OMS v1.2  07/21/05/IM CN-LMLN/Saccade Enable/LN FPh Gen/event timer1 ==
  note: Resettable
      | Event Timer
  note: This block is an RESETTABLE EVENT TIMER.  It outputs a spike of unit height xx milliseconds
      | (set by "timer value") after it detects an event ( i.e a TRAILING edge which represents the end of a
      |  saccadic pulse)
  note: (Init input: 0)
  note: (FF init state: Q=0)
  note: (Init input: 0)
  note: Therefore, an event first RESETS and then SETS the flip-flop.
  note: The "OR" gate allows either of these conditions to reset the circuit.  The delay before the
      | "S" input of the flip-flop prevents both "S" and "R" from being set simultaneously, because
      | this would put the flip-flop in an undefined state.
  note: The real trick here is understanding how to reload the countdown.
      | It resets if either of two conditions is met:
  note: It has TWO modes: 1) Event resettable and 2) Event Non-resettable
  note: In 1), Any event (leading or trailing edge) will reset the counter so that it
      | counts down from the end trailing edge) of that event.
  note: 1) The count reaches its limit (set in "timer value") -- Both case 1) and 2)
  note: 2) A new event (leading or trailing edge) is detected. -- Only case 1)
  note: In 2) Subsequent events DO NOT reset the counter; it only resets when it
      | reaches zero
  _PG : Inport
  _timer value (port) : Inport  Port=2
  1 msec : TransportDelay  DelayTime=.001
  Clock : Clock
      settings: Decimation=10
  Latch1 : simulink_extras/Flip Flops/S-R Flip-Flop  SystemSampleTime=-1  initial_condition=0
  Logical Operator : Logic  Operator=OR  Inputs=3
  Logical Operator1 : Logic
  Logical Operator2 : Logic
  Relational Operator : RelationalOperator  InputSameDT=on
  SampHold?1 : Subsystem
      mask Display: disp('S&H\n(S=L)\n(H=H)')
  Sum : Sum  Inputs=+-  SaturateOnIntegerOverflow=on  InputSameDT=on
  Terminator : Terminator
  event resettable? : Constant  Orientation=up
  leading edge detect : Subsystem
      mask Display: disp('Leading\nEdge Det')
  loop breaker : Memory  Orientation=left
  trailing edge detect : Subsystem
      mask Display: disp('Trailing\nEdge Det')
  out_1 : Outport  InitialOutput=0
  wires:
  _timer value (port)/1 -> Relational Operator/2
  1 msec/1 -> Latch1/1
  Logical Operator/1 -> Latch1/2
  SampHold?1/1(output) -> Sum/2
  Relational Operator/1 -> loop breaker/1, out_1/1
  _PG/1 -> trailing edge detect/1(in_1), leading edge detect/1(in_1)
  Clock/1 -> Sum/1, SampHold?1/1(Input)
  Sum/1 -> Relational Operator/1
  Latch1/1 -> SampHold?1/2(S/H?)
  loop breaker/1 -> Logical Operator/3
  Logical Operator1/1 -> Logical Operator/1
  trailing edge detect/1(out_1) -> Logical Operator1/1, 1 msec/1
  Logical Operator2/1 -> Logical Operator/2
  leading edge detect/1(out_1) -> Logical Operator2/1
  event resettable?/1 -> Logical Operator2/2, Logical Operator1/2
  Latch1/2 -> Terminator/1

== system OMSv1_2x/OMS v1.2  07/21/05/IM CN-LMLN/Saccade Enable/LN FPh Gen/leading edge detect ==
  note: leading edge detection
  in_1 : Inport
  Abs : Abs  SaturateOnIntegerOverflow=on
  Derivative : Derivative
  Relational Operator : RelationalOperator  Operator===  InputSameDT=on
  Sign : Signum
  Threshold 1 : Constant
  out_1 : Outport  InitialOutput=0
  wires:
  in_1/1 -> Abs/1
  Relational Operator/1 -> out_1/1
  Threshold 1/1 -> Relational Operator/2
  Sign/1 -> Relational Operator/1
  Derivative/1 -> Sign/1
  Abs/1 -> Derivative/1

== system OMSv1_2x/OMS v1.2  07/21/05/IM CN-LMLN/Saccade Enable/Ret FB sample/Boolify ==
  In1 : Inport
  Abs2 : Abs  SaturateOnIntegerOverflow=on
  direction1 : Signum
  Out1 : Outport  InitialOutput=0
  wires:
  Abs2/1 -> direction1/1
  In1/1 -> Abs2/1
  direction1/1 -> Out1/1
